simulink model "AdaptiveBacksteppingProva"  (R2019b)
settings: Solver=ode23s  StartTime=0.0  StopTime=25  RelTol=1e-3  AbsTol=1e-6
undefined symbols (not defined in the file): a0, a1, a2, a3, dq0, Kd_endEff, lambda, parameter, Pi0, q0, R, x_endEff_D
libraries: simulink x1
settings Model: Creator=ariannagasparri  LastModifiedBy=ariannagasparri

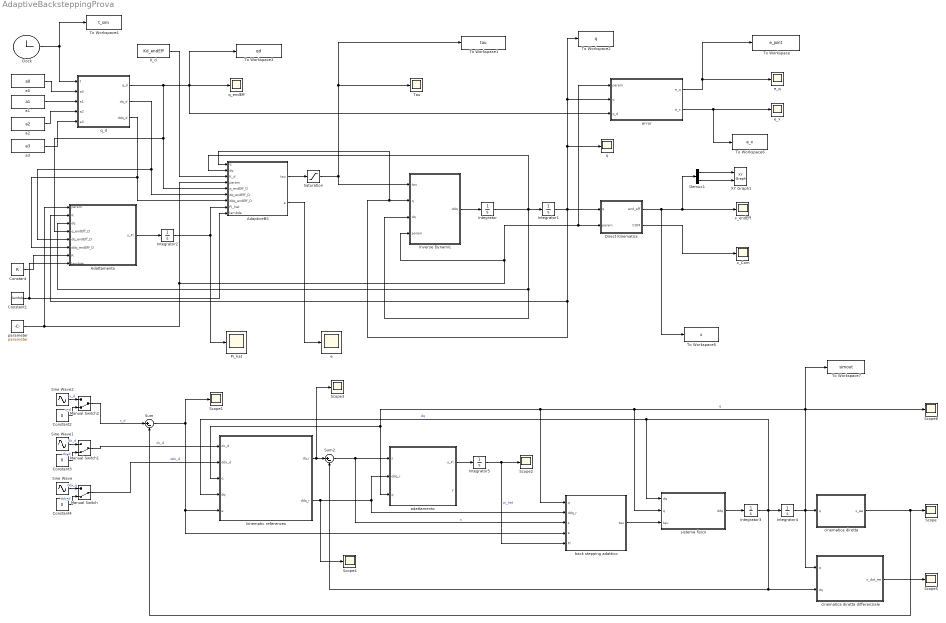
== system AdaptiveBacksteppingProva ==
  AdaptiveBS : MATLAB Function  TreatAsAtomicUnit=on
  Adattamento : MATLAB Function  TreatAsAtomicUnit=on
  Clock : Clock
  Constant : Constant  Value=R
  Constant1 : Constant  Value=lambda
  Constant2 : Constant  Value=0
  Constant3 : Constant  Value=0
  Constant4 : Constant  Value=0
  Demux1 : Demux  Outputs=3
  "Direct Kinematics " : MATLAB Function  TreatAsAtomicUnit=on
  Integrator : Integrator  InitialCondition=q0
  Integrator1 : Integrator  InitialCondition=dq0
  Integrator2 : Integrator  InitialCondition=Pi0
  Integrator3 : Integrator
  Integrator4 : Integrator  InitialCondition=-pi/8
  Integrator5 : Integrator  InitialCondition=[1; 9.81]*0.8
  "Inverse Dynamic " : MATLAB Function  TreatAsAtomicUnit=on
  K_d : Constant  Value=Kd_endEff
  Manual Switch : ManualSwitch  CurrentSetting=0
  Manual Switch1 : ManualSwitch  CurrentSetting=0
  Manual Switch2 : ManualSwitch  CurrentSetting=0
  Pi_hat : Scope
  Saturation : Saturate  UpperLimit=35000  LowerLimit=-35000
  Scope{,1..6} (7 alike) : Scope
  Sine Wave : Sin  Amplitude=0.8  Phase=pi  SampleTime=0
  Sine Wave1 : Sin  Amplitude=0.8  Phase=pi/2  SampleTime=0
  Sine Wave2 : Sin  Amplitude=0.8  SampleTime=0
  Sum : Sum  Inputs=|+-
  Sum2 : Sum  Inputs=|+-
  Tau : Scope
  To Workspace : ToWorkspace  VariableName=e_joint  SaveFormat=Structure With Time  SampleTime=-1
      settings: Save2DSignal=2-D array (concatenate along first dimension)
  To Workspace1 : ToWorkspace  VariableName=tau  SaveFormat=Structure With Time  SampleTime=-1
  To Workspace2 : ToWorkspace  VariableName=q  SaveFormat=Structure With Time  SampleTime=-1
  To Workspace3 : ToWorkspace  VariableName=qd  SaveFormat=Structure With Time  SampleTime=-1
  To Workspace4 : ToWorkspace  VariableName=t_sim  SaveFormat=Structure With Time  SampleTime=-1
  To Workspace5 : ToWorkspace  VariableName=x  SaveFormat=Structure With Time  SampleTime=-1
  To Workspace6 : ToWorkspace  VariableName=e_x  SaveFormat=Structure With Time  SampleTime=-1
  To Workspace7 : ToWorkspace  VariableName=simout  SaveFormat=Timeseries  SampleTime=-1
  XY Graph1 : simulink/Sinks/XY Graph  xmin=x_endEff_D(1)-2  xmax=x_endEff_D(1)+2  ymin=x_endEff_D(3)-2  ymax=x_endEff_D(3)+2  st=-1
  a0 : Constant  Value=a0
  a1 : Constant  Value=a1
  a2 : Constant  Value=a2
  a3 : Constant  Value=a3
  adattamento : MATLAB Function  TreatAsAtomicUnit=on
  back stepping adattivo : MATLAB Function  TreatAsAtomicUnit=on
  cinematica diretta : MATLAB Function  TreatAsAtomicUnit=on
  cinematica diretta differenziale : MATLAB Function  TreatAsAtomicUnit=on
  e : Scope
  e_q : Scope
  e_x : Scope
  error : MATLAB Function  TreatAsAtomicUnit=on
  kinematic references : Subsystem
  "parameter " : Constant  Value=parameter
  q : Scope
  q_d : MATLAB Function  TreatAsAtomicUnit=on
  q_endEff : Scope
  sistema fisico : MATLAB Function  TreatAsAtomicUnit=on
  x_Com : Scope
  x_endEff : Scope
  wires:
  error/2(e_x) -> To Workspace6/1, e_x/1
  Demux1/3 -> XY Graph1/2
  "Direct Kinematics "/1(end_eff) -> To Workspace5/1, Demux1/1, x_endEff/1
  Clock/1 -> q_d/1(t), To Workspace4/1
  "Direct Kinematics "/2(COM) -> x_Com/1
  Demux1/1 -> XY Graph1/1
  AdaptiveBS/2(e) -> e/1
  "Inverse Dynamic "/1(ddq) -> Integrator/1
  a3/1 -> q_d/5(a3)
  "parameter "/1 -> Adattamento/1(param), AdaptiveBS/4(param), "Inverse Dynamic "/4(param), error/1(param), "Direct Kinematics "/2(param)
  a0/1 -> q_d/2(a0)
  a2/1 -> q_d/4(a2)
  q_d/3(ddq_d) -> Adattamento/6(ddq_endEff_D), AdaptiveBS/7(ddq_endEff_D)
  Saturation/1 -> To Workspace1/1, Tau/1, "Inverse Dynamic "/1(tau)
  Integrator1/1 -> "Direct Kinematics "/1(q), To Workspace2/1, error/2(q), q/1, Adattamento/2(q), AdaptiveBS/1(q), "Inverse Dynamic "/2(q)
  Integrator2/1 -> Pi_hat/1, AdaptiveBS/8(Pi_hat)
  q_d/1(q_d) -> Adattamento/4(q_endEff_D), AdaptiveBS/5(q_endEff_D), error/3(q_d), To Workspace3/1, q_endEff/1
  Integrator/1 -> AdaptiveBS/2(dq), Adattamento/3(dq), "Inverse Dynamic "/3(dq), Integrator1/1
  Constant/1 -> Adattamento/7(R)
  q_d/2(dq_d) -> Adattamento/5(dq_endEff_D), AdaptiveBS/6(dq_endEff_D)
  a1/1 -> q_d/3(a1)
  Adattamento/1(u_Pi) -> Integrator2/1
  error/1(e_q) -> To Workspace/1, e_q/1
  Constant1/1 -> AdaptiveBS/9(lambda), Adattamento/8(lambda)
  AdaptiveBS/1(tau) -> Saturation/1
  K_d/1 -> AdaptiveBS/3(K_d)
  sistema fisico/1(ddq) -> Integrator3/1
  Constant3/1 -> Manual Switch1/2  "dx_d"
  back stepping adattivo/1(tau) -> sistema fisico/3(tau)
  Manual Switch/1 -> kinematic references/2(ddx_d)  "ddx_d"
  kinematic references/2(ddq_r) -> Scope4/1, back stepping adattivo/2(ddq_r), adattamento/2(ddq_r)
  Constant4/1 -> Manual Switch/2  "ddx_d"
  adattamento/1(u_Pi) -> Integrator5/1
  Constant2/1 -> Manual Switch2/2  "x_d"
  Sum/1 -> back stepping adattivo/4(e), kinematic references/5("e "), Scope1/1
  Integrator5/1 -> back stepping adattivo/5(Pi), Scope2/1  "pi_hat"
  cinematica diretta/1(x_ee) -> Sum/2, Scope/1
  Sum2/1 -> back stepping adattivo/3(s), adattamento/1(s)  "s"
  cinematica diretta differenziale/1(x_dot_ee) -> Scope5/1
  Sine Wave/1 -> Manual Switch/1  "ddx_q"
  Manual Switch1/1 -> kinematic references/1(dx_d)  "dx_d"
  Manual Switch2/1 -> Sum/1  "x_d"
  Sine Wave1/1 -> Manual Switch1/1  "dx_d"
  kinematic references/1(dq_r) -> Scope3/1, Sum2/1
  Integrator4/1 -> To Workspace7/1, sistema fisico/2(q), back stepping adattivo/1(q), adattamento/3(q), kinematic references/3(q), Scope6/1, cinematica diretta/1(q), cinematica diretta differenziale/1(q)  "q"
  Sine Wave2/1 -> Manual Switch2/1  "x_d"
  Integrator3/1 -> Integrator4/1, cinematica diretta differenziale/2(dq), Sum2/2, sistema fisico/1(dq), kinematic references/4(dq)  "dq"

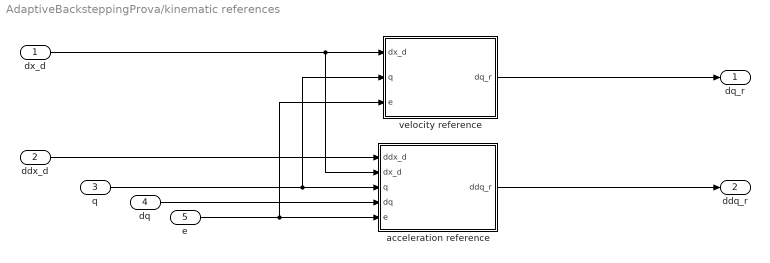
== system AdaptiveBacksteppingProva/kinematic references ==
  dx_d : Inport
  ddx_d : Inport  Port=2
  q : Inport  Port=3
  dq : Inport  Port=4
  "e " : Inport  Port=5
  acceleration reference : MATLAB Function  TreatAsAtomicUnit=on
  velocity reference : MATLAB Function  TreatAsAtomicUnit=on
  dq_r : Outport
  ddq_r : Outport  Port=2
  wires:
  dx_d/1 -> acceleration reference/2(dx_d), velocity reference/1(dx_d)
  ddx_d/1 -> acceleration reference/1(ddx_d)
  "e "/1 -> acceleration reference/5(e), velocity reference/3(e)
  q/1 -> velocity reference/2(q), acceleration reference/3(q)
  acceleration reference/1(ddq_r) -> ddq_r/1
  velocity reference/1(dq_r) -> dq_r/1
  dq/1 -> acceleration reference/4(dq)

== matlab function AdaptiveBacksteppingProva/Direct Kinematics  ==
  data: q input; end_eff output; param input; COM output
function [end_eff, COM] = DirectK(q,param)

    [Pcom, Etip, ~, ~, ~, ~, ~, ~, ~] =  forwardKinematics(param, q);
    
    end_eff = Etip(1:3, 4);
    COM = Pcom;
    
end

== matlab function AdaptiveBacksteppingProva/Inverse Dynamic  ==
  data: tau input; q input; dq input; ddq output; param input
function ddq = inverseDynamic(tau, q, dq, param)

    B = B_fun(param, q);
    C = C_fun(param, q, dq);
    G = G_fun(param, q);
    
    ddq = pinv(B)*(tau - G - C*dq);

end

== matlab function AdaptiveBacksteppingProva/AdaptiveBS ==
  data: q input; tau output; dq input; K_d input; param input; q_endEff_D input; dq_endEff_D input; e output; ddq_endEff_D input; Pi_hat input; lambda input
function [tau, e]  = x_now(q, dq, K_d, param, q_endEff_D, dq_endEff_D, ddq_endEff_D, Pi_hat, lambda)

    Y = Y_fun(param, q, dq, ddq_endEff_D);
    
    [Pcom, Etip] = forwardKinematics(param, q_endEff_D);
    x_endEff_D = Etip(1:3, 4);
    [Pcom, Etip] = forwardKinematics(param, q);
    x = Etip(1:3, 4);
    J = JacobianEndEff(param, q);
    dx_endEff_D = J * dq_endEff_D;
    dx = J * dq;

    e = x_endEff_D - x;
    de = dx_endEff_D - dx;
    
    s = pinv(J) * (de + lambda * e);
    
    tau = Y * Pi_hat + K_d * s + J' * e;

end

== matlab function AdaptiveBacksteppingProva/adattamento ==
  data: s input; ddq_r input; q input; u_Pi output; Y output
function [u_Pi, Y] = adattamento(s, ddq_r, q)

% Pi =  [l^2*m ;  g*l*m ]

R = diag([10 10]);
Y = [ddq_r, cos(q)];

u_Pi = inv(R) * Y' * s;

== matlab function AdaptiveBacksteppingProva/error ==
  data: param input; q input; e_q output; q_d input; e_x output
function [e_q, e_x]  = error(param, q, q_d)
    

    [~, Etip, ~, ~, ~, ~, ~, ~, ~] =  forwardKinematics(param, q);
    [~, Etip_d, ~, ~, ~, ~, ~, ~, ~] =  forwardKinematics(param, q_d);  

    e_x = Etip_d(1:3,4) - Etip(1:3,4);

    e_q = q_d - q;
    
end

== matlab function AdaptiveBacksteppingProva/q_d ==
  data: t input; q_d output; dq_d output; ddq_d output; a0 input; a1 input; a2 input; a3 input
function [q_d, dq_d, ddq_d] = desiderable_q(t, a0, a1, a2, a3)

    [q_d, dq_d, ddq_d] = vettoreq(a0, a1, a2, a3, t);
    
end

== matlab function AdaptiveBacksteppingProva/Adattamento ==
  data: param input; q input; dq input; q_endEff_D input; dq_endEff_D input; ddq_endEff_D input; u_Pi output; R input; lambda input
function u_Pi = adattamento(param, q, dq, q_endEff_D, dq_endEff_D, ddq_endEff_D, R, lambda)

    Y = Y_fun(param, q, dq, ddq_endEff_D);

    [Pcom, Etip] = forwardKinematics(param, q_endEff_D);
    x_endEff_D = Etip(1:3,4);
    [Pcom, Etip] = forwardKinematics(param, q);
    x = Etip(1:3,4);
    J = JacobianEndEff(param, q);
    dx_endEff_D = J * dq_endEff_D;
    dx = J * dq;

    e = x_endEff_D - x;
    de = dx_endEff_D - dx;

    s = pinv(J) * (de + lambda * e);

    u_Pi = pinv(R) * Y' * s;

end

== matlab function AdaptiveBacksteppingProva/back stepping adattivo ==
  data: q input; tau output; ddq_r input; s input; e input; Pi input
function tau = back_stepping_adattivo(q, ddq_r, s, e, Pi)


tau = 0;
% m = 1;      % kg massa del pendolo
l = 1;      % m lunghezza del pendolo
% g  = 9.81;  % kg*m/s^2 acc di gravita'

% Pi =  [l^2*m ;  g*l*m ]

% Pi =  [1 ;  9,81 ]

Kd = 2;

J = l*cos(q);   % Jacobian

tau = Pi(1)*ddq_r + Pi(2)*cos(q) + Kd*s + J.'*e;

== matlab function AdaptiveBacksteppingProva/cinematica diretta ==
  data: q input; x_ee output
function x_ee = cinematica_diretta(q)

l = 1;      % m lunghezza del pendolo

x_ee = l*sin(q);

== matlab function AdaptiveBacksteppingProva/cinematica diretta differenziale ==
  data: q input; x_dot_ee output; dq input
function x_dot_ee = cinematica_diff_diretta(q, dq)

l = 1;          % m lunghezza del pendolo

J = l*cos(q);   % Jacobian

x_dot_ee = J*dq;

== matlab function AdaptiveBacksteppingProva/kinematic references/acceleration reference ==
  data: ddx_d input; dx_d input; q input; dq input; ddq_r output; e input
function ddq_r = acc_ref(ddx_d, dx_d, q, dq, e)
ddq_r = 0;

l = 1;      % m lunghezza del pendolo

J = l*cos(q);   % Jacobian
dJ = -l*sin(q); % Derivative of Jacobian

Lambda = 5;

ddq_r = inv(J)*(ddx_d + Lambda*dx_d - Lambda*J*dq) - inv(J)*(dJ*dq)*inv(J)*(dx_d + Lambda*e);

== matlab function AdaptiveBacksteppingProva/kinematic references/velocity reference ==
  data: dx_d input; q input; dq_r output; e input
function dq_r = vel_ref(dx_d, q, e)
dq_r = 0;

l = 1;      % m lunghezza del pendolo

J = l*cos(q);   % Jacobian

Lambda = 5;

dq_r = inv(J)*(dx_d + Lambda*e);

== matlab function AdaptiveBacksteppingProva/sistema fisico ==
  data: dq input; q input; ddq output; tau input
function ddq = dyn(dq, q, tau)

m = 1;      % kg massa del pendolo
l = 1;      % m lunghezza del pendolo
g  = 9.81;  % kg*m/s^2 acc di gravita'

ddq = (tau - g*l*m*cos(q))/(l^2*m);
